simulink model "SOC_conversion_Load_Switcher"  (R2022b)
settings: Solver=VariableStepAuto  StartTime=0.0  StopTime=15  RelTol=1e-3
libraries: spsIdealSwitchLib x4, simulink x1
settings Model: Creator=Haposan  LastModifiedBy=Haposan

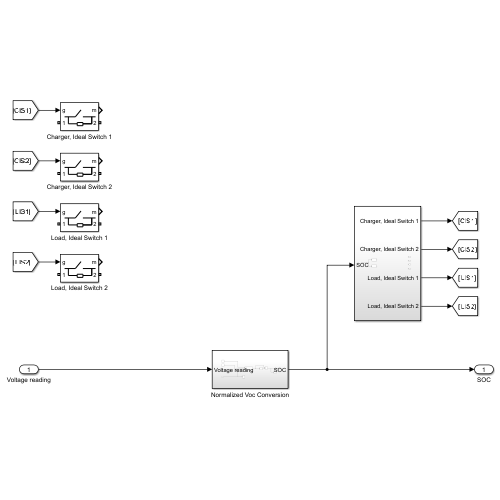
[thumbnail: Simulink's stored preview of the top-level diagram]
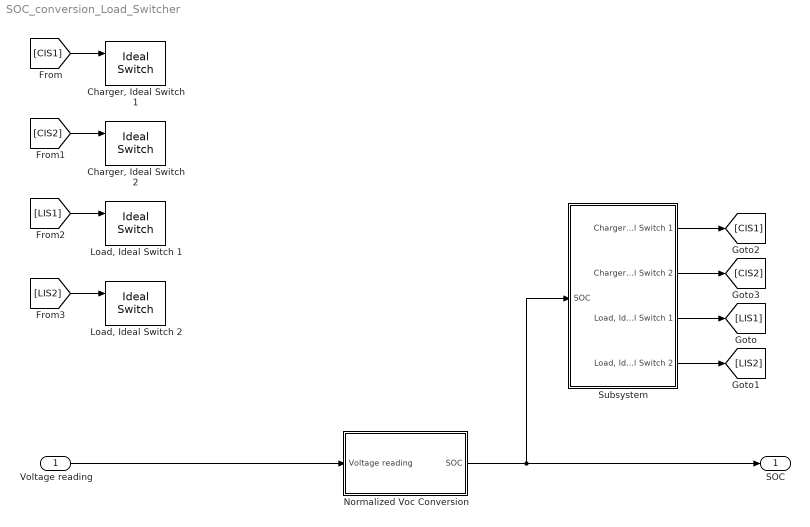
== system SOC_conversion_Load_Switcher ==
  Voltage reading : Inport
  "Charger, Ideal Switch 1" : spsIdealSwitchLib/Ideal Switch  Ron=0.001  Lon=0  IC=0  Rs=1e5  Cs=inf  Measurements=on
  "Charger, Ideal Switch 2" : spsIdealSwitchLib/Ideal Switch  Ron=0.001  Lon=0  IC=0  Rs=1e5  Cs=inf  Measurements=on
  "Load, Ideal Switch 1" : spsIdealSwitchLib/Ideal Switch  Ron=0.001  Lon=0  IC=0  Rs=1e5  Cs=inf  Measurements=on
  "Load, Ideal Switch 2" : spsIdealSwitchLib/Ideal Switch  Ron=0.001  Lon=0  IC=0  Rs=1e5  Cs=inf  Measurements=on
  Normalized Voc Conversion : Subsystem
  Subsystem : Subsystem
  SOC : Outport
  wires:
  Voltage reading/1 -> Normalized Voc Conversion/1(Voltage reading)
  Normalized Voc Conversion/1(SOC) -> Subsystem/1(SOC), SOC/1
  Subsystem/1("Charger, Ideal Switch 1") -> [CIS1]
  Subsystem/2("Charger, Ideal Switch 2") -> [CIS2]
  Subsystem/3("Load, Ideal Switch 1") -> [LIS1]
  Subsystem/4("Load, Ideal Switch 2") -> [LIS2]
  [CIS1] -> "Charger, Ideal Switch 1"/1
  [CIS2] -> "Charger, Ideal Switch 2"/1
  [LIS1] -> "Load, Ideal Switch 1"/1
  [LIS2] -> "Load, Ideal Switch 2"/1

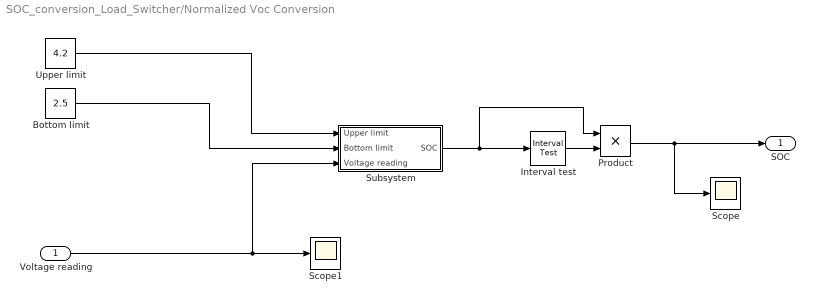
== system SOC_conversion_Load_Switcher/Normalized Voc Conversion ==
  Voltage reading : Inport
  Bottom limit : Constant  Value=2.5
  Interval test : simulink/Logic and Bit Operations/Interval Test  IntervalClosedRight=on  uplimit=100  IntervalClosedLeft=on  lowlimit=0  OutDataTypeStr=boolean
  Product : Product
  Scope : Scope
  Scope1 : Scope
  Subsystem : Subsystem
  Upper limit : Constant  Value=4.2
  SOC : Outport
  wires:
  Voltage reading/1 -> Subsystem/3(Voltage reading), Scope1/1
  Upper limit/1 -> Subsystem/1(Upper limit)
  Product/1 -> SOC/1, Scope/1
  Subsystem/1(SOC) -> Product/1, Interval test/1
  Interval test/1 -> Product/2
  Bottom limit/1 -> Subsystem/2(Bottom limit)

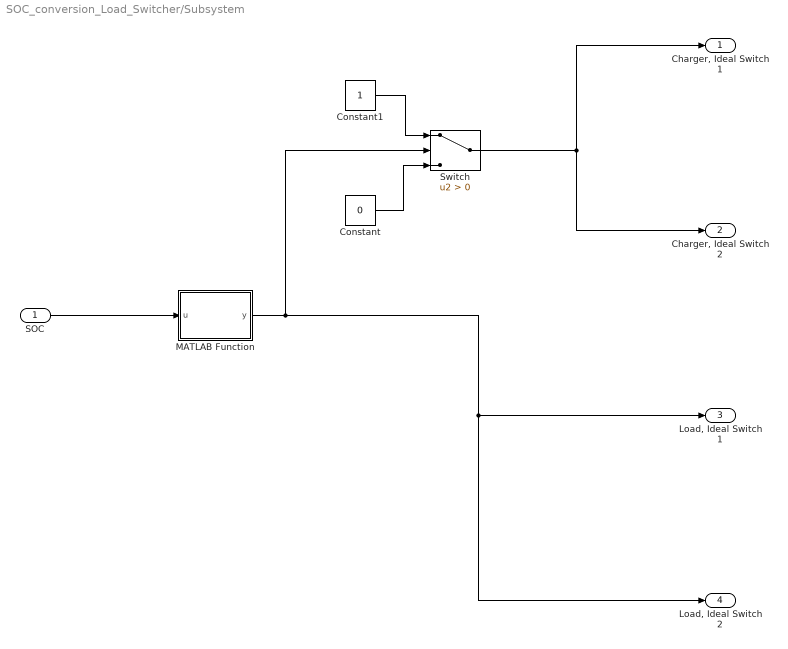
== system SOC_conversion_Load_Switcher/Subsystem ==
  SOC : Inport
  Constant : Constant  Value=0
  Constant1 : Constant
  MATLAB Function : MATLAB Function  TreatAsAtomicUnit=on
  Switch : Switch  Criteria=u2 > Threshold  SaturateOnIntegerOverflow=off  InputSameDT=off
  "Charger, Ideal Switch 1" : Outport
  "Charger, Ideal Switch 2" : Outport  Port=2
  "Load, Ideal Switch 1" : Outport  Port=3
  "Load, Ideal Switch 2" : Outport  Port=4
  wires:
  SOC/1 -> MATLAB Function/1(u)
  MATLAB Function/1(y) -> Switch/2, "Load, Ideal Switch 2"/1, "Load, Ideal Switch 1"/1
  Constant/1 -> Switch/3
  Constant1/1 -> Switch/1
  Switch/1 -> "Charger, Ideal Switch 2"/1, "Charger, Ideal Switch 1"/1

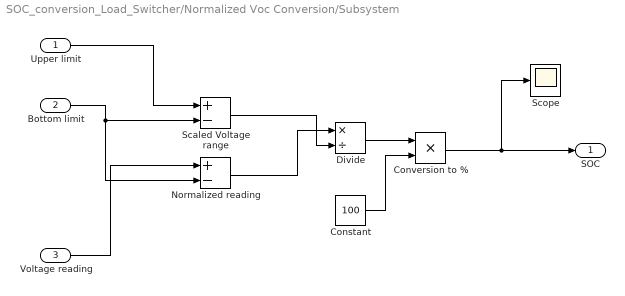
== system SOC_conversion_Load_Switcher/Normalized Voc Conversion/Subsystem ==
  Upper limit : Inport
  Bottom limit : Inport  Port=2
  Voltage reading : Inport  Port=3
  Constant : Constant  Value=100
  Conversion to % : Product
  Divide : Product  Inputs=*/
  Normalized reading : Sum  Inputs=+-
  Scaled Voltage range : Sum  Inputs=+-
  Scope : Scope
  SOC : Outport
  wires:
  Upper limit/1 -> Scaled Voltage range/1
  Bottom limit/1 -> Normalized reading/2, Scaled Voltage range/2
  Voltage reading/1 -> Normalized reading/1
  Normalized reading/1 -> Divide/1
  Scaled Voltage range/1 -> Divide/2
  Divide/1 -> Conversion to %/1
  Constant/1 -> Conversion to %/2
  Conversion to %/1 -> Scope/1, SOC/1

== matlab function SOC_conversion_Load_Switcher/Subsystem/MATLAB Function ==
  data: u input; y output
function y = switch_output(u)
y = 0
    if u >= 99.5
        y = 1;
    elseif u <= 0.05
        y = 0;
    else
        y = y;  % keep the previous value of y
    end
end
